simulink model "cordic_atan_cosim"  (Simulink 6.4)
settings: Solver=FixedStepDiscrete  SolverMode=SingleTasking  StartTime=0.0  StopTime=1.5e-1  RelTol=1e-3
undefined symbols (not defined in the file or in its folder): pipeline_prec
libraries: modelsimlib x1, simulink x1
settings Model: LastModifiedBy=Administrador

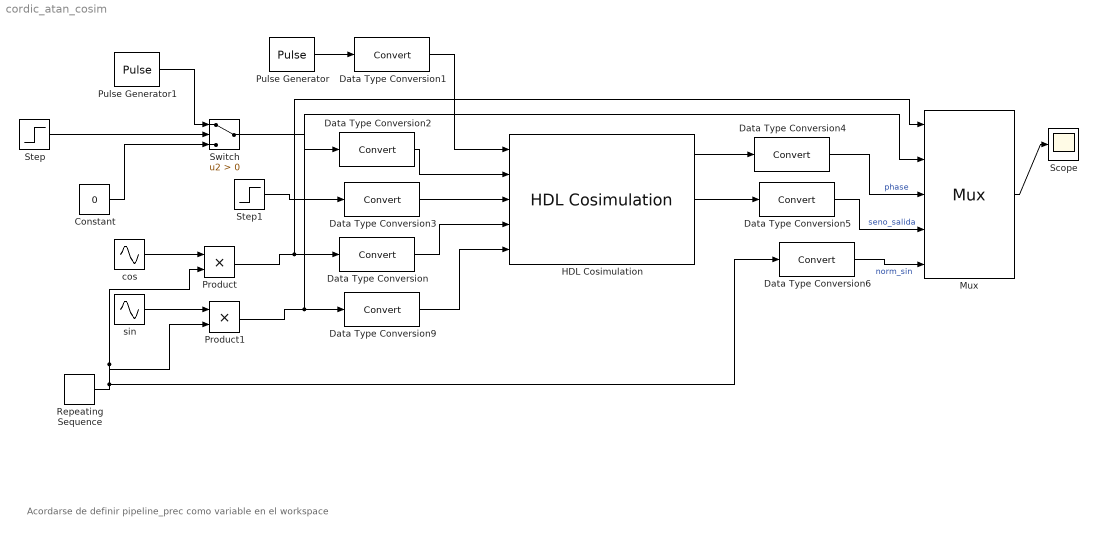
== system cordic_atan_cosim ==
  note: Acordarse de definir pipeline_prec como variable en el workspace
  Constant : Constant  Value=0  OutDataType=sfix(16)  ConRadixGroup=Use specified scaling  OutScaling=2^0  SampleTime=-1  FramePeriod=inf
  Data Type Conversion : DataTypeConversion  OutDataTypeMode=Specify via dialog  OutScaling=2^(-pipeline_prec)  RndMeth=Nearest  SampleTime=1e-5  SaturateOnIntegerOverflow=on
  Data Type Conversion1 : DataTypeConversion  OutDataTypeMode=boolean
  Data Type Conversion2 : DataTypeConversion  OutDataTypeMode=boolean
  Data Type Conversion3 : DataTypeConversion  OutDataTypeMode=boolean
  Data Type Conversion4 : DataTypeConversion
  Data Type Conversion5 : DataTypeConversion
  Data Type Conversion6 : DataTypeConversion
  Data Type Conversion9 : DataTypeConversion  OutDataTypeMode=Specify via dialog  OutScaling=2^(-pipeline_prec)  RndMeth=Nearest  SampleTime=1e-5  SaturateOnIntegerOverflow=on
  HDL Cosimulation : modelsimlib/HDL Cosimulation  DialogController=modelsimddg.CoSim  DialogControllerArgs=DataTag0  PortPaths=/cordic_atan/clk;/cordic_atan/run;/cordic_atan/rst;/cordic_atan/x;/cordic_atan/y;/cordic_atan/angle;/cordic_atan/modu;/cordic_atan/done  PortModes=[1 1 1 1 1 2 2 2 ]  PortTimes=[1,1,1,1,1,1e-5,1e-5,1]  PortSigns=[-1 -1 -1 -1 -1 1 1 -1 ]  PortFracLengths=[0,0,0,0,0,pipeline_prec,pipeline_prec,0]  CommLocal=on  CommSharedMemory=off  CommPortNumber=4449  CommShowInfo=on  ClockModes=[]  ClockTimes=[]  TclPreSimCommand="echo \"Running Simulink Cosimulation block.\""  TclPostSimCommand="echo \"done\""  TimingMode=s  TimingScaleFactor=1  idxCellArray={'UNUSED_VAR'}
  Mux : Mux  Inputs=5
  Product : Product  RndMeth=Zero
  Product1 : Product  RndMeth=Zero
  Pulse Generator : DiscretePulseGenerator  PulseType=Time based  Period=1/(1e6)  PulseWidth=50
  Pulse Generator1 : DiscretePulseGenerator  PulseType=Time based  Period=0.1e-3  PulseWidth=2
  Repeating Sequence : simulink/Sources/Repeating Sequence  SystemSampleTime=-1  rep_seq_t=[0:1:8] .* 1/50  rep_seq_y=[0 0.2 0.3 0.5 0.8 1.0 1.6 2 -1]
  Scope : Scope
      settings: YMin=-3.5  YMax=3.5  MaxDataPoints=500000  Decimation=3
  Step : Step  Time=4*(1/1e6)
  Step1 : Step  Time=6*(1/1e6)  Before=1  After=0
  Switch : Switch  Criteria=u2 > Threshold  RndMeth=Nearest  ZeroCross=off  SampleTime=1e-7
  cos : Sin  Frequency=2*pi*50  Phase=pi/2
  sin : Sin  Frequency=2*pi*50
  wires:
  Data Type Conversion/1 -> HDL Cosimulation/4
  Pulse Generator/1 -> Data Type Conversion1/1
  Data Type Conversion1/1 -> HDL Cosimulation/1
  Switch/1 -> Data Type Conversion2/1
  Data Type Conversion2/1 -> HDL Cosimulation/2
  Step1/1 -> Data Type Conversion3/1
  Data Type Conversion3/1 -> HDL Cosimulation/3
  Constant/1 -> Switch/3
  Step/1 -> Switch/2
  Pulse Generator1/1 -> Switch/1
  Mux/1 -> Scope/1
  HDL Cosimulation/1 -> Data Type Conversion4/1
  HDL Cosimulation/2 -> Data Type Conversion5/1
  Data Type Conversion9/1 -> HDL Cosimulation/5
  cos/1 -> Product/1
  Product/1 -> Data Type Conversion/1, Mux/1
  sin/1 -> Product1/1
  Product1/1 -> Data Type Conversion9/1, Mux/2
  Repeating Sequence/1 -> Product/2, Product1/2, Data Type Conversion6/1
  Data Type Conversion4/1 -> Mux/3  "phase"
  Data Type Conversion5/1 -> Mux/4  "seno_salida"
  Data Type Conversion6/1 -> Mux/5  "norm_sin"
